simulink model "test2_px4"  (R2022b)
settings: Solver=ode4  StartTime=0.0  StopTime=inf  FixedStep=0.004  RelTol=1e-3
undefined symbols (not defined in the file or in its folder): Earth, Payload, WGS84
libraries: uavmavlinklib x5, px4MAVLinkBridgelib x2, shared6dof x1, aerolibtransform2 x1, test_px4 x1, instrumentlib x1
settings Model: Creator=User  LastModifiedBy=User

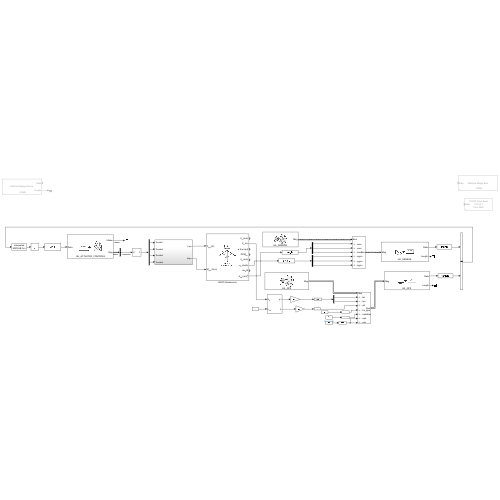
[thumbnail: Simulink's stored preview of the top-level diagram]
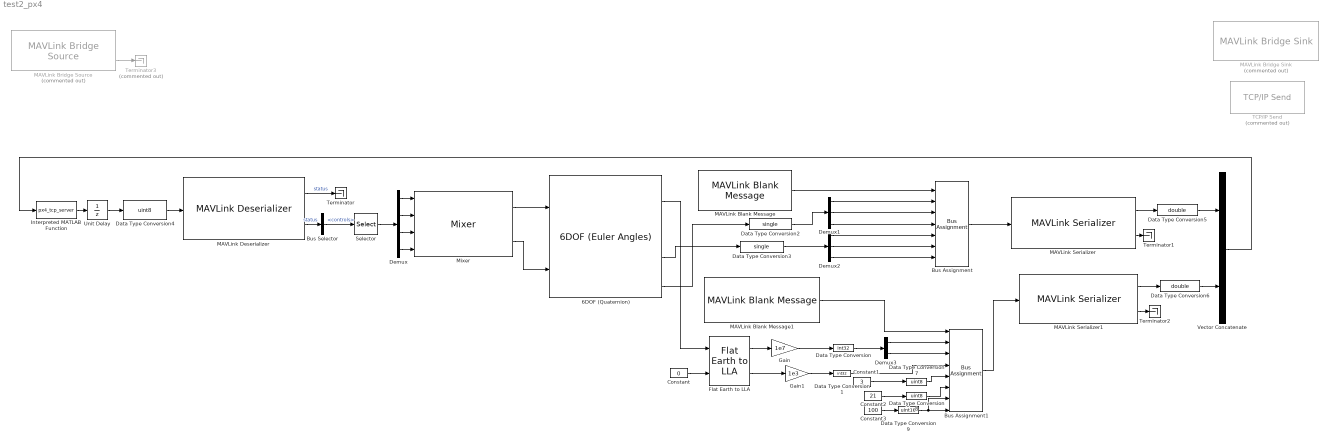
== system test2_px4 ==
  6DOF (Quaternion) : shared6dof/6DOF (Euler Angles)  units=Metric (MKS)  mtype=Fixed  rep=Quaternion  xme_0=[0 0 0]  Vm_0=[0 0 0]  eul_0=[0 0 0]  pm_0=[0 0 0]  mass_0=1.0  mass_e=0.5  mass_f=2.0  inertia=eye(3)  inertia_e=eye(3)  inertia_f=2*eye(3)  k_quat=1.0  vre_flag=on  abi_flag=off  aMode=0  xme_statename=''  Vm_statename=''  eul_statename=''  quat_statename=''  pm_statename=''  mass_statename=''
      settings: LibrarySourceBlock=aerolib6dof2/6DOF (Quaternion)
  Bus Assignment : BusAssignment  AssignedSignals=Payload.xacc,Payload.yacc,Payload.zacc,Payload.xgyro,Payload.ygyro,Payload.zgyro
  Bus Assignment1 : BusAssignment  AssignedSignals=Payload.lat,Payload.lon,Payload.alt,Payload.fix_type,Payload.satellites_visible,Payload.eph,Payload.epv
  Bus Selector : BusSelector  OutputSignals=Payload.controls
  Constant : Constant  Value=0
  Constant1 : Constant  Value=3
  Constant2 : Constant  Value=21
  Constant3 : Constant  Value=100
  Data Type Conversion : DataTypeConversion  OutDataTypeStr=int32  SaturateOnIntegerOverflow=off  RndMeth=Floor
  Data Type Conversion1 : DataTypeConversion  OutDataTypeStr=int32  SaturateOnIntegerOverflow=off  RndMeth=Floor
  Data Type Conversion2 : DataTypeConversion  OutDataTypeStr=single  SaturateOnIntegerOverflow=off  RndMeth=Floor
  Data Type Conversion3 : DataTypeConversion  OutDataTypeStr=single  SaturateOnIntegerOverflow=off  RndMeth=Floor
  Data Type Conversion4 : DataTypeConversion  OutDataTypeStr=uint8  SaturateOnIntegerOverflow=off  RndMeth=Floor
  Data Type Conversion5 : DataTypeConversion  OutDataTypeStr=double  SaturateOnIntegerOverflow=off  RndMeth=Floor
  Data Type Conversion6 : DataTypeConversion  OutDataTypeStr=double  SaturateOnIntegerOverflow=off  RndMeth=Floor
  Data Type Conversion7 : DataTypeConversion  OutDataTypeStr=uint8  SaturateOnIntegerOverflow=off  RndMeth=Floor
  Data Type Conversion8 : DataTypeConversion  OutDataTypeStr=uint8  SaturateOnIntegerOverflow=off  RndMeth=Floor
  Data Type Conversion9 : DataTypeConversion  OutDataTypeStr=uint16  SaturateOnIntegerOverflow=off  RndMeth=Floor
  Demux : Demux
  Demux1 : Demux  Outputs=3
  Demux2 : Demux  Outputs=3
  Demux3 : Demux  Outputs=2
  Flat Earth to LLA : aerolibtransform2/Flat Earth to LLA  units=Metric (MKS)  ptype=Earth (WGS84)  F=1/298.257223563  R=6378137  refPosPort=off  LL0=[0 10]  psi=0
  Gain : Gain  Gain=1e7
  Gain1 : Gain  Gain=1e3
  Interpreted MATLAB Function : MATLABFcn  MATLABFcn=px4_tcp_server
  MAVLink Blank Message : uavmavlinklib/MAVLink Blank Message  dialectSource=Select from standard MAVLink dialects  dialect=common.xml  dialectCustom=common.xml  version=2  messageType=HIL_SENSOR  SystemID=1  ComponentID=1  SampleTime=inf
  MAVLink Blank Message1 : uavmavlinklib/MAVLink Blank Message  dialectSource=Select from standard MAVLink dialects  dialect=common.xml  dialectCustom=common.xml  version=2  messageType=HIL_GPS  SystemID=1  ComponentID=1  SampleTime=inf
  MAVLink Bridge Sink : px4MAVLinkBridgelib/MAVLink Bridge Sink  Commented=on  PixhawkSerialPorttemp=Specify manually  PixhawkSerialPortManually=COM4  FieldTable={ 'TCP', '0.0.0.0', '4560' }
  MAVLink Bridge Source : px4MAVLinkBridgelib/MAVLink Bridge Source  Commented=on  PixhawkSerialPorttemp=Specify manually  PixhawkSerialPortManually=COM4  dataLength=1024  FieldTable={ 'TCP', '0.0.0.0', '4560' }  SampleTime=0.004
  MAVLink Deserializer : uavmavlinklib/MAVLink Deserializer  dialectSource=Select from standard MAVLink dialects  dialect=common.xml  dialectCustom=common.xml  version=2  messageType=HIL_ACTUATOR_CONTROLS  inputDataLength=off  SystemIDFilter=off  systemID=1  ComponentIDFilter=off  componentID=1  queueMsg=off  queueMsgSize=50  dropNum=off
  MAVLink Serializer : uavmavlinklib/MAVLink Serializer  dialectSource=Select from standard MAVLink dialects  dialect=common.xml  dialectCustom=common.xml  version=2  messageType=HIL_SENSOR
  MAVLink Serializer1 : uavmavlinklib/MAVLink Serializer  dialectSource=Select from standard MAVLink dialects  dialect=common.xml  dialectCustom=common.xml  version=2  messageType=HIL_GPS
  Mixer : test_px4/Mixer  SystemSampleTime=-1  VariantActivationTime=update diagram  Latency=0  AutoFrameSizeCalculation=off
  Selector : Selector  NumberOfDimensions=2  InputPortWidth=4  IndexOptions=Select all,Index vector (dialog)  Indices=[1:4],[1:4]  OutputSizes=1,1
  TCP/IP Send : instrumentlib/TCP//IP Send  Commented=on  Host=127.0.0.1  Port=4560  ByteOrder=big-endian  EnableBlockingMode=on  Timeout=10  TransferDelay=on  SimulateUsing=Interpreted execution
  Terminator : Terminator
  Terminator1 : Terminator
  Terminator2 : Terminator
  Terminator3 : Terminator  Commented=on
  Unit Delay : UnitDelay  SampleTime=0.004  HasFrameUpgradeWarning=on
  Vector Concatenate : Concatenate
  wires:
  Mixer/2 -> 6DOF (Quaternion)/2
  Mixer/1 -> 6DOF (Quaternion)/1
  Interpreted MATLAB Function/1 -> Unit Delay/1
  MAVLink Serializer/1 -> Data Type Conversion5/1
  MAVLink Deserializer/2 -> Bus Selector/1  "status"
  MAVLink Deserializer/1 -> Terminator/1  "status"
  Demux/1 -> Mixer/1
  Demux/4 -> Mixer/4
  Demux/2 -> Mixer/2
  Demux/3 -> Mixer/3
  Bus Selector/1 -> Selector/1  "<controls>"
  Selector/1 -> Demux/1
  MAVLink Serializer1/1 -> Data Type Conversion6/1
  MAVLink Blank Message/1 -> Bus Assignment/1
  Bus Assignment/1 -> MAVLink Serializer/1
  Demux1/1 -> Bus Assignment/2
  Demux1/3 -> Bus Assignment/4
  Demux1/2 -> Bus Assignment/3
  6DOF (Quaternion)/8 -> Data Type Conversion2/1
  Demux2/1 -> Bus Assignment/5
  Demux2/2 -> Bus Assignment/6
  Demux2/3 -> Bus Assignment/7
  6DOF (Quaternion)/6 -> Data Type Conversion3/1
  MAVLink Blank Message1/1 -> Bus Assignment1/1
  6DOF (Quaternion)/2 -> Flat Earth to LLA/1
  Constant/1 -> Flat Earth to LLA/2
  Flat Earth to LLA/1 -> Gain/1
  Demux3/1 -> Bus Assignment1/2
  Demux3/2 -> Bus Assignment1/3
  Flat Earth to LLA/2 -> Gain1/1
  Bus Assignment1/1 -> MAVLink Serializer1/1
  MAVLink Serializer/2 -> Terminator1/1
  MAVLink Serializer1/2 -> Terminator2/1
  Gain/1 -> Data Type Conversion/1
  Data Type Conversion/1 -> Demux3/1
  Gain1/1 -> Data Type Conversion1/1
  Data Type Conversion1/1 -> Bus Assignment1/4
  Data Type Conversion2/1 -> Demux1/1
  Data Type Conversion3/1 -> Demux2/1
  MAVLink Bridge Source/2 -> Terminator3/1
  Data Type Conversion4/1 -> MAVLink Deserializer/1
  Vector Concatenate/1 -> Interpreted MATLAB Function/1
  Data Type Conversion5/1 -> Vector Concatenate/1
  Data Type Conversion6/1 -> Vector Concatenate/2
  Unit Delay/1 -> Data Type Conversion4/1
  Constant1/1 -> Data Type Conversion7/1
  Constant2/1 -> Data Type Conversion8/1
  Constant3/1 -> Data Type Conversion9/1
  Data Type Conversion7/1 -> Bus Assignment1/5
  Data Type Conversion8/1 -> Bus Assignment1/6
  Data Type Conversion9/1 -> Bus Assignment1/7, Bus Assignment1/8
